simulink model "mqsls_sim_6dof_actual"  (R2024b)
settings: configuration reference "prj_default_config" (kept outside this file)
StartFcn:
  | run('control_init.m');
settings Model: Creator=yangyu  LastModifiedBy=yangyu
settings ConfigSetRef: SourceName=prj_default_config  SourceLocation=Base Workspace

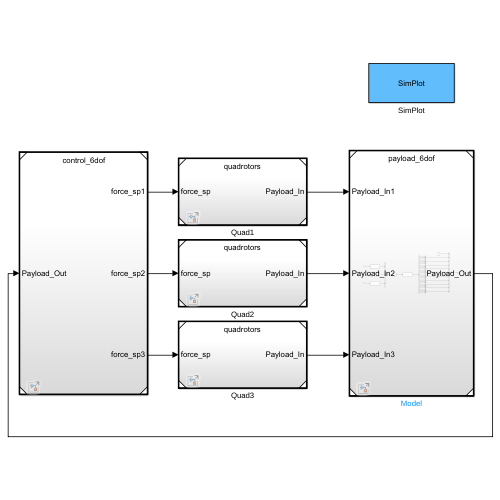
[thumbnail: Simulink's stored preview of the top-level diagram]
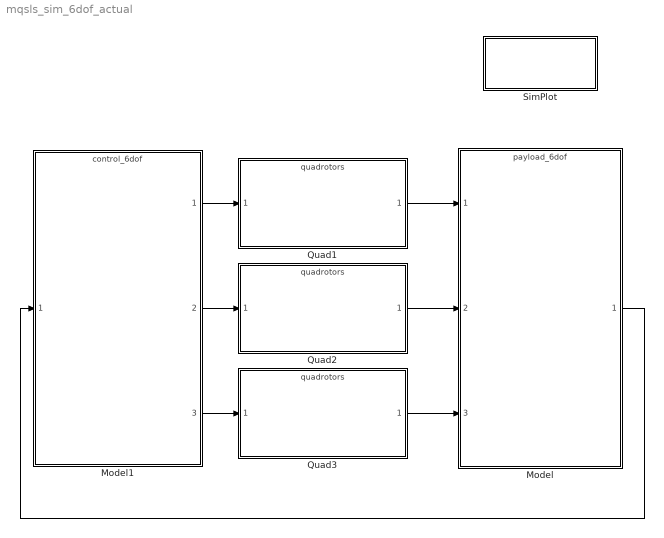
== system mqsls_sim_6dof_actual ==
  Model : ModelReference  ModelNameDialog=payload_6dof.slx  SimulationMode=Normal  ModelReferenceVersion=1.103
  Model1 : ModelReference  ModelNameDialog=control_6dof.slx  SimulationMode=Normal  ModelReferenceVersion=1.421
  Quad1 : ModelReference  ModelNameDialog=quadrotors.slx  SimulationMode=Normal  ModelReferenceVersion=1.84
  Quad2 : ModelReference  ModelNameDialog=quadrotors.slx  SimulationMode=Normal  ModelReferenceVersion=1.84
  Quad3 : ModelReference  ModelNameDialog=quadrotors.slx  SimulationMode=Normal  ModelReferenceVersion=1.84
  SimPlot : Subsystem
      settings: OpenFcn=run('simplot.m');
      mask Display: disp('SimPlot');
  wires:
  Quad1/1 -> Model/1
  Model1/1 -> Quad1/1
  Quad2/1 -> Model/2
  Model1/2 -> Quad2/1
  Quad3/1 -> Model/3
  Model1/3 -> Quad3/1
  Model/1 -> Model1/1

== system mqsls_sim_6dof_actual/SimPlot ==
